simulink library "lib_right_angle_side_length_calculator"  (R2023a)
settings: Solver=VariableStepAuto  StartTime=0.0  StopTime=10.0  RelTol=1e-3
libraries: lib_conversion x3, simulink x2
settings Model: Creator=cav2ofo  LastModifiedBy=lenovo
settings OptimizationCC: ReuseModelBlockBuffer=off

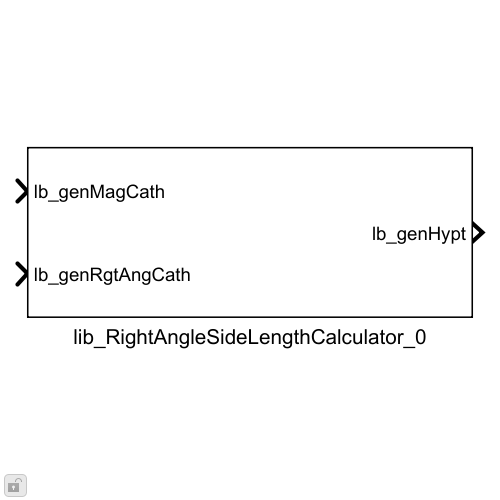
[thumbnail: Simulink's stored preview of the top-level diagram]
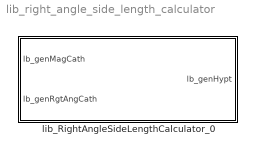
== system lib_right_angle_side_length_calculator ==
  lib_RightAngleSideLengthCalculator_0 : Subsystem  mask{lb_parLktSize=512, lb_parOutpDataType=Inherit: Inherit via back propagation}
      mask prompts: lb_parLktSize "Look-up table size:"; lb_parOutpDataType "Output data type:"
      mask init:
      | lb_parLktSizeNum = str2double(lb_parLktSize);
      | lb_parLktInpData = linspace(0,1,lb_parLktSizeNum).^2;
      | lb_parLktOutpData = sqrt(1-lb_parLktInpData);
      mask TypeOptions lb_parLktSize: 32 | 64 | 128 | 256 | 512 | 1024 | 2048 | 4096
      mask DialogControl DescGroupVar Prompt: WEIFU motor control library
      mask DialogControl DescTextVar Prompt: Right triangle right side length calculator
      mask DialogControl Container3 Prompt: Data type

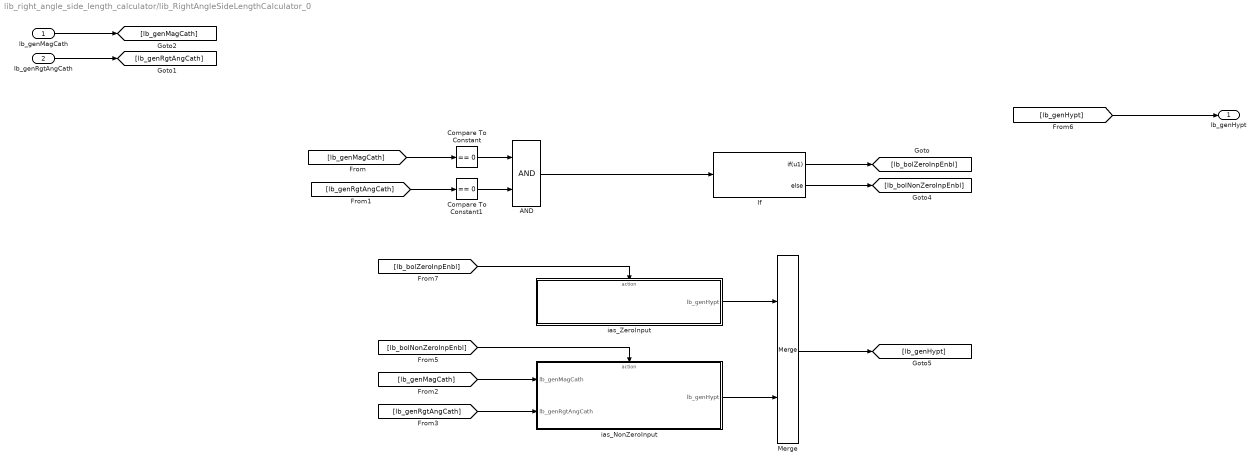
== system lib_right_angle_side_length_calculator/lib_RightAngleSideLengthCalculator_0 ==
  lb_genMagCath : Inport
  lb_genRgtAngCath : Inport  Port=2
  AND : Logic  AllPortsSameDT=off  OutDataTypeStr=boolean
  Compare To Constant : simulink/Logic and Bit Operations/Compare To Constant  relop===  const=0  OutDataTypeStr=boolean
  Compare To Constant1 : simulink/Logic and Bit Operations/Compare To Constant  relop===  const=0  OutDataTypeStr=boolean
  If : If  IfExpression=u1
  Merge : Merge
  ias_NonZeroInput : Subsystem  TreatAsAtomicUnit=on
  ias_ZeroInput : Subsystem  TreatAsAtomicUnit=on
  lb_genHypt : Outport
  wires:
  [lb_genHypt] -> lb_genHypt/1
  AND/1 -> If/1
  If/1 -> [lb_bolZeroInpEnbl]
  If/2 -> [lb_bolNonZeroInpEnbl]
  [lb_bolZeroInpEnbl] -> ias_ZeroInput/Action
  [lb_bolNonZeroInpEnbl] -> ias_NonZeroInput/Action
  ias_ZeroInput/1(lb_genHypt) -> Merge/1
  ias_NonZeroInput/1(lb_genHypt) -> Merge/2
  Merge/1 -> [lb_genHypt]
  lb_genRgtAngCath/1 -> [lb_genRgtAngCath]
  lb_genMagCath/1 -> [lb_genMagCath]
  [lb_genMagCath] -> Compare To Constant/1
  [lb_genRgtAngCath] -> Compare To Constant1/1
  Compare To Constant1/1 -> AND/2
  Compare To Constant/1 -> AND/1
  [lb_genMagCath] -> ias_NonZeroInput/1(lb_genMagCath)
  [lb_genRgtAngCath] -> ias_NonZeroInput/2(lb_genRgtAngCath)

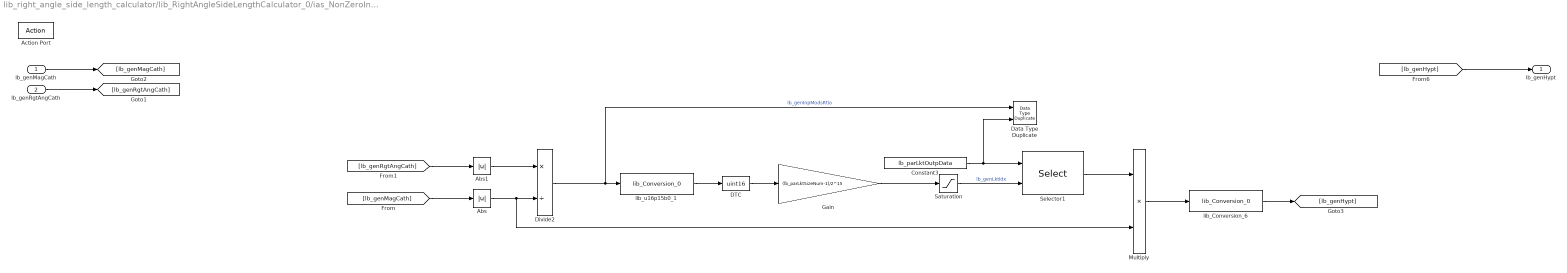
== system lib_right_angle_side_length_calculator/lib_RightAngleSideLengthCalculator_0/ias_NonZeroInput ==
  lb_genMagCath : Inport
  lb_genRgtAngCath : Inport  Port=2
  Action Port : ActionPort
  Abs : Abs  RndMeth=Simplest  SaturateOnIntegerOverflow=off
  Abs1 : Abs  RndMeth=Simplest  SaturateOnIntegerOverflow=off
  Constant3 : Constant  Value=lb_parLktOutpData  OutDataTypeStr=Inherit: Inherit via back propagation
  DTC : DataTypeConversion  OutDataTypeStr=uint16  ConvertRealWorld=Stored Integer (SI)  RndMeth=Simplest  SaturateOnIntegerOverflow=off
  Data Type Duplicate : DataTypeDuplicate
  Divide2 : Product  Inputs=*/  OutDataTypeStr=Inherit: Inherit via back propagation  RndMeth=Simplest
  Gain : Gain  Gain=(lb_parLktSizeNum-1)/2^15  OutDataTypeStr=uint16  RndMeth=Simplest
  Multiply : Product  OutDataTypeStr=Inherit: Inherit via back propagation  RndMeth=Simplest
  Saturation : Saturate  UpperLimit=lb_parLktSizeNum-1  LowerLimit=0
  Selector1 : Selector  IndexMode=Zero-based  InputPortWidth=lb_parLktSizeNum  IndexOptions=Index vector (port)  Indices=[1 3]  OutputSizes=1
  lib_Conversion_6 : lib_conversion/lib_Conversion_0  lb_parDataType=lb_parOutpDataType  lb_parOutpMaxVal=[]  lb_parOutpMinVal=[]  lb_parSatFlag=off
  lib_u16p15b0_1 : lib_conversion/lib_Conversion_0  lb_parDataType=fixdt(0,16,2^-15,0)  lb_parOutpMaxVal=[]  lb_parOutpMinVal=[]  lb_parSatFlag=off
  lb_genHypt : Outport
  wires:
  [lb_genHypt] -> lb_genHypt/1
  lb_genRgtAngCath/1 -> [lb_genRgtAngCath]
  lb_genMagCath/1 -> [lb_genMagCath]
  [lb_genRgtAngCath] -> Abs1/1
  Divide2/1 -> lib_u16p15b0_1/1, Data Type Duplicate/1  "lb_genInpModsRtio"
  lib_u16p15b0_1/1 -> DTC/1
  DTC/1 -> Gain/1
  Gain/1 -> Saturation/1
  Constant3/1 -> Data Type Duplicate/2, Selector1/1
  Selector1/1 -> Multiply/1
  Multiply/1 -> lib_Conversion_6/1
  lib_Conversion_6/1 -> [lb_genHypt]
  [lb_genMagCath] -> Abs/1
  Saturation/1 -> Selector1/2  "lb_genLktIdx"
  Abs/1 -> Multiply/2, Divide2/2
  Abs1/1 -> Divide2/1

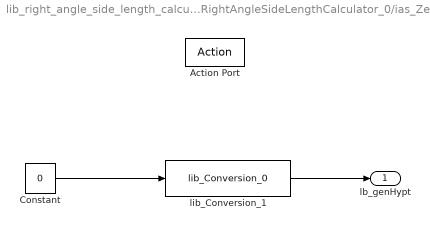
== system lib_right_angle_side_length_calculator/lib_RightAngleSideLengthCalculator_0/ias_ZeroInput ==
  Action Port : ActionPort
  Constant : Constant  Value=0  OutDataTypeStr=Inherit: Inherit via back propagation
  lib_Conversion_1 : lib_conversion/lib_Conversion_0  lb_parDataType=lb_parOutpDataType  lb_parOutpMaxVal=[]  lb_parOutpMinVal=[]  lb_parSatFlag=off
  lb_genHypt : Outport
  wires:
  Constant/1 -> lib_Conversion_1/1
  lib_Conversion_1/1 -> lb_genHypt/1
